simulink model "envelope_analysis_simulink2"  (R2020a)
settings: Solver=FixedStepDiscrete  StartTime=0.0  StopTime=inf  RelTol=1e-3
values from neighbouring files (symbols this model uses):
  fs = 48e3    (= 48000)    [bearing_sim.m]    (also in decimation.m; demodulation.m)
libraries: dspfdesign x6, dspsigops x2, dspsrcs4 x1
settings Model: PacingRate=0.100000  Creator=holge  LastModifiedBy=holge
settings SolverCC: AutoInsertRateTranBlk=on
settings DataIOCC: LimitDataPoints=on  SaveOutput=off  SignalLogging=off  SaveTime=off
settings OptimizationCC: LifeSpan=inf  SimCompilerOptimization=on
settings DebuggingCC: AlgebraicLoopMsg=error  SingleTaskRateTransMsg=error  AllowSymbolicDim=off  SFUnexpectedBacktrackingDiag=warning  SFNoUnconditionalDefaultTransitionDiag=warning  SFExecutionAtInitializationDiag=none  ArithmeticOperatorsInVariantConditions=warning
settings SFSimCC: SimUseLocalCustomCode=off  CustomCodeUndefinedFunction=UseInterfaceOnly
settings RTWCC: RTWUseLocalCustomCode=off
settings CodeAppCC: StateflowObjectComments=on
settings GRTTargetCC: TargetLangStandard=C89/C90 (ANSI)
settings ConfigComp: CovMetricSettings=dw  CovHtmlReporting=on  CovSaveCumulativeToWorkspaceVar=on  CovSaveSingleToWorkspaceVar=on  CovExternalEMLEnable=off  CovSFcnEnable=off

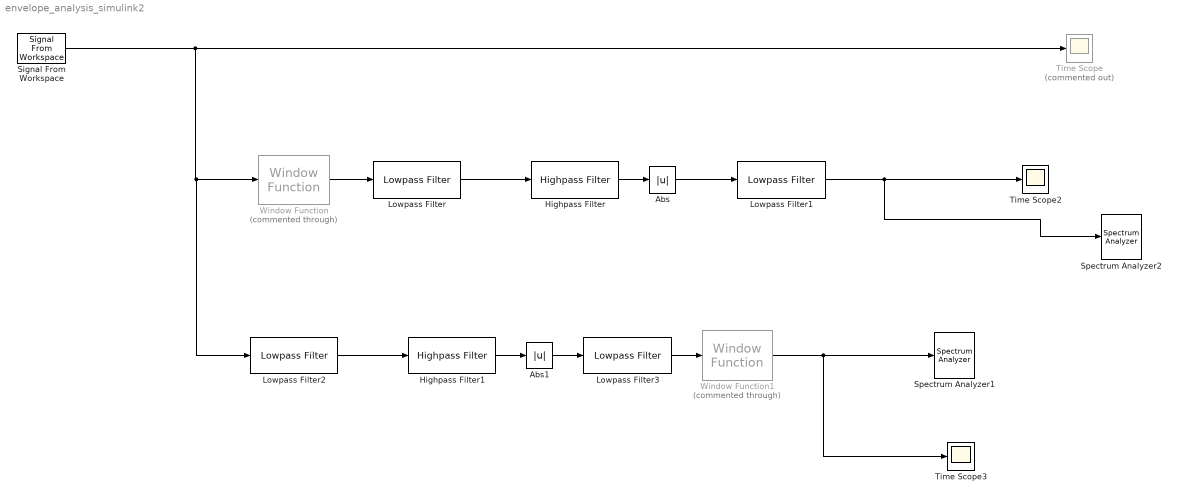
== system envelope_analysis_simulink2 ==
  Abs : Abs
  Abs1 : Abs
  Highpass Filter : dspfdesign/Highpass Filter  FilterType=FIR  DesignForMinimumOrder=on  FilterOrder=50  StopbandFrequency=100  PassbandFrequency=500  StopbandAttenuation=80  PassbandRipple=0.1  InheritSampleRate=off  SampleRate=fs  SimulateUsing=Interpreted execution  roundingMode=Floor  coeffsDataTypeStr=fixdt(1,16)
  Highpass Filter1 : dspfdesign/Highpass Filter  FilterType=IIR  DesignForMinimumOrder=on  FilterOrder=50  StopbandFrequency=800  PassbandFrequency=1000  StopbandAttenuation=80  PassbandRipple=0.1  InheritSampleRate=on  SampleRate=fs  SimulateUsing=Interpreted execution  roundingMode=Floor  coeffsDataTypeStr=fixdt(1,16)
  Lowpass Filter : dspfdesign/Lowpass Filter  FilterType=FIR  DesignForMinimumOrder=on  FilterOrder=50  PassbandFrequency=20e3  StopbandFrequency=22e3  PassbandRipple=0.1  StopbandAttenuation=80  InheritSampleRate=off  SampleRate=48000  SimulateUsing=Interpreted execution  roundingMode=Floor  coeffsDataTypeStr=fixdt(1,16)
  Lowpass Filter1 : dspfdesign/Lowpass Filter  FilterType=FIR  DesignForMinimumOrder=on  FilterOrder=50  PassbandFrequency=1e3  StopbandFrequency=1.2e3  PassbandRipple=0.1  StopbandAttenuation=80  InheritSampleRate=on  SampleRate=44100  SimulateUsing=Interpreted execution  roundingMode=Floor  coeffsDataTypeStr=fixdt(1,16)
  Lowpass Filter2 : dspfdesign/Lowpass Filter  FilterType=FIR  DesignForMinimumOrder=on  FilterOrder=50  PassbandFrequency=20e3  StopbandFrequency=22e3  PassbandRipple=0.1  StopbandAttenuation=80  InheritSampleRate=off  SampleRate=48000  SimulateUsing=Interpreted execution  roundingMode=Floor  coeffsDataTypeStr=fixdt(1,16)
  Lowpass Filter3 : dspfdesign/Lowpass Filter  FilterType=FIR  DesignForMinimumOrder=on  FilterOrder=50  PassbandFrequency=1000  StopbandFrequency=1.2e3  PassbandRipple=0.1  StopbandAttenuation=50  InheritSampleRate=on  SampleRate=44100  SimulateUsing=Interpreted execution  roundingMode=Floor  coeffsDataTypeStr=fixdt(1,16)
  Signal From Workspace : dspsrcs4/Signal From Workspace  X=xBper  Ts=1/fs  nsamps=1024  OutputAfterFinalValue=Cyclic repetition  ignoreOrWarnInputAndFrameLengths=off  OutputFrames=off
  Spectrum Analyzer1 : SpectrumAnalyzer
  Spectrum Analyzer2 : SpectrumAnalyzer
  Time Scope : Scope  Commented=on
  Time Scope2 : Scope
  Time Scope3 : Scope
  Window Function : dspsigops/Window Function  Commented=through  winmode=Apply window to input  wintype=Hanning  sampmode=Continuous  samptime=1  N=64  Rs=50  beta=10  winsamp=Periodic  UserWindow=hamming  OptParams=off  UserParams={'symmetric'}  dataType=double  isSigned=on  wordLen=16  udDataType=sfix(16)  fracBitsMode=Best precision  numFracBits=15  roundingMode=Floor  overflowMode=off  numSidelobes=4  sidelobeLevel=-30
      settings: SourceProductBaseCode=DS
  Window Function1 : dspsigops/Window Function  Commented=through  winmode=Apply window to input  wintype=Hanning  sampmode=Continuous  samptime=1  N=64  Rs=50  beta=10  winsamp=Periodic  UserWindow=hamming  OptParams=off  UserParams={'symmetric'}  dataType=double  isSigned=on  wordLen=16  udDataType=sfix(16)  fracBitsMode=Best precision  numFracBits=15  roundingMode=Floor  overflowMode=off  numSidelobes=4  sidelobeLevel=-30
      settings: SourceProductBaseCode=DS
  wires:
  Lowpass Filter/1 -> Highpass Filter/1
  Highpass Filter/1 -> Abs/1
  Abs/1 -> Lowpass Filter1/1
  Window Function/1 -> Lowpass Filter/1
  Lowpass Filter1/1 -> Spectrum Analyzer2/1, Time Scope2/1
  Signal From Workspace/1 -> Lowpass Filter2/1, Window Function/1, Time Scope/1
  Lowpass Filter2/1 -> Highpass Filter1/1
  Abs1/1 -> Lowpass Filter3/1
  Lowpass Filter3/1 -> Window Function1/1
  Window Function1/1 -> Time Scope3/1, Spectrum Analyzer1/1
  Highpass Filter1/1 -> Abs1/1
